simulink model "InverterComm2015"  (Simulink 8.1)
settings: Solver=ode45  StartTime=0.0  StopTime=10.0  RelTol=1e-3
libraries: simulink x24
settings Model: Creator=Brian  LastModifiedBy=Brian
settings DataIOCC: SignalLoggingSaveFormat=Dataset
settings OptimizationCC: ExpressionDepthLimit=128
settings DebuggingCC: FcnCallInpInsideContextMsg=EnableAllAsError
settings GRTTargetCC: CombineOutputUpdateFcns=on  GRTInterface=off

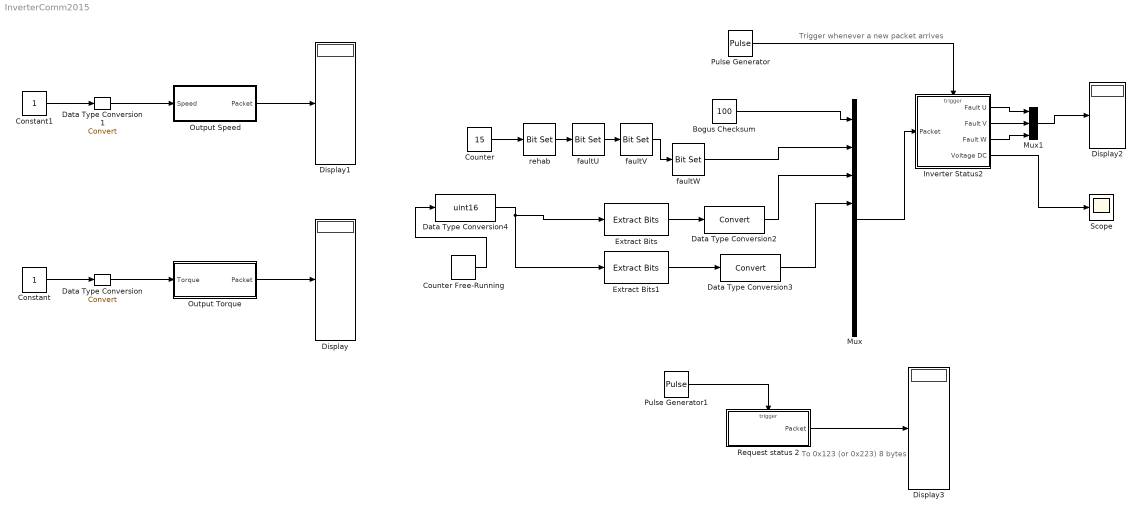
== system InverterComm2015 ==
  note: To 0x123 (or 0x223)
      | 8 bytes
  note: Trigger whenever a new packet arrives
  Bogus Checksum : Constant  Value=100  OutDataTypeStr=uint8
  Constant : Constant
  Constant1 : Constant
  Counter : Constant  Value=15  OutDataTypeStr=uint8
  Counter Free-Running : simulink/Sources/Counter Free-Running  NumBits=4  tsamp=-1
  Data Type Conversion : DataTypeConversion
  Data Type Conversion1 : DataTypeConversion
  Data Type Conversion2 : DataTypeConversion  ConvertRealWorld=Stored Integer (SI)
  Data Type Conversion3 : DataTypeConversion  ConvertRealWorld=Stored Integer (SI)
  Data Type Conversion4 : DataTypeConversion  OutDataTypeStr=uint16  ConvertRealWorld=Stored Integer (SI)
  Display{,1..3} (4 alike) : Display
      settings: Format=hex (Stored Integer)
  Extract Bits : simulink/Logic and Bit Operations/Extract Bits  bitsToExtract=Upper half  numBits=8  bitIdxRange=[0 7]  outScalingMode=Preserve fixed-point scaling
  Extract Bits1 : simulink/Logic and Bit Operations/Extract Bits  bitsToExtract=Lower half  numBits=8  bitIdxRange=[0 7]  outScalingMode=Preserve fixed-point scaling
  Inverter Status2 : Subsystem
  Mux : Mux  Inputs=8
  Mux1 : Mux  Inputs=3
  Output Speed : Subsystem
  Output Torque : Subsystem
  Pulse Generator : DiscretePulseGenerator  PulseType=Time based  Period=.1  PulseWidth=5
  Pulse Generator1 : DiscretePulseGenerator  PulseType=Time based  Period=.1  PulseWidth=5
  Request status 2 : Subsystem
  Scope : Scope
  faultU : simulink/Logic and Bit Operations/Bit Set  iBit=5
  faultV : simulink/Logic and Bit Operations/Bit Set  iBit=6
  faultW : simulink/Logic and Bit Operations/Bit Set  iBit=7
  rehab : simulink/Logic and Bit Operations/Bit Set  iBit=4
  wires:
  Output Torque/1(Packet) -> Display/1
  Constant/1 -> Data Type Conversion/1
  Data Type Conversion/1 -> Output Torque/1(Torque)
  Output Speed/1(Packet) -> Display1/1
  Constant1/1 -> Data Type Conversion1/1
  Data Type Conversion1/1 -> Output Speed/1(Speed)
  Pulse Generator/1 -> Inverter Status2/Trigger
  Mux/1 -> Inverter Status2/1(Packet)
  Bogus Checksum/1 -> Mux/1
  Counter/1 -> rehab/1
  rehab/1 -> faultU/1
  faultU/1 -> faultV/1
  faultV/1 -> faultW/1
  faultW/1 -> Mux/2
  Extract Bits/1 -> Data Type Conversion2/1
  Extract Bits1/1 -> Data Type Conversion3/1
  Counter Free-Running/1 -> Data Type Conversion4/1
  Data Type Conversion2/1 -> Mux/3
  Data Type Conversion3/1 -> Mux/4
  Inverter Status2/1(Fault U) -> Mux1/1
  Inverter Status2/2(Fault V) -> Mux1/2
  Inverter Status2/3(Fault W) -> Mux1/3
  Mux1/1 -> Display2/1
  Inverter Status2/4(Voltage DC) -> Scope/1
  Data Type Conversion4/1 -> Extract Bits1/1, Extract Bits/1
  Request status 2/1(Packet) -> Display3/1
  Pulse Generator1/1 -> Request status 2/Trigger

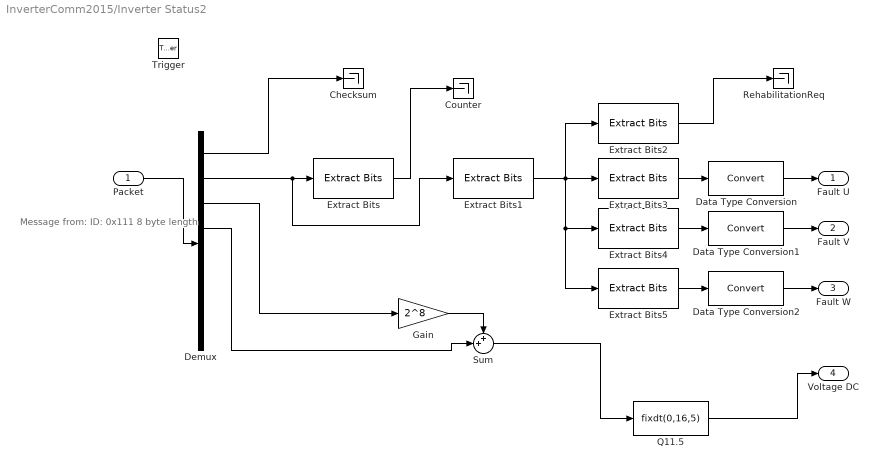
== system InverterComm2015/Inverter Status2 ==
  note: Message from:
      | ID: 0x111
      | 8 byte length
  Packet : Inport  OutDataTypeStr=uint8  PortDimensions=8
  Trigger : TriggerPort  PortDimensions=1
  Checksum : Terminator
  Counter : Terminator
  Data Type Conversion : DataTypeConversion
  Data Type Conversion1 : DataTypeConversion
  Data Type Conversion2 : DataTypeConversion
  Demux : Demux  Outputs=8
  Extract Bits : simulink/Logic and Bit Operations/Extract Bits  bitsToExtract=Lower half  numBits=8  bitIdxRange=[0 7]  outScalingMode=Treat bit field as an integer
  Extract Bits1 : simulink/Logic and Bit Operations/Extract Bits  bitsToExtract=Upper half  numBits=8  bitIdxRange=[0 7]  outScalingMode=Treat bit field as an integer
  Extract Bits2 : simulink/Logic and Bit Operations/Extract Bits  bitsToExtract=Range of bits  numBits=8  bitIdxRange=[0 0]  outScalingMode=Treat bit field as an integer
  Extract Bits3 : simulink/Logic and Bit Operations/Extract Bits  bitsToExtract=Range of bits  numBits=8  bitIdxRange=[1 1]  outScalingMode=Treat bit field as an integer
  Extract Bits4 : simulink/Logic and Bit Operations/Extract Bits  bitsToExtract=Range of bits  numBits=8  bitIdxRange=[2 2]  outScalingMode=Treat bit field as an integer
  Extract Bits5 : simulink/Logic and Bit Operations/Extract Bits  bitsToExtract=Range of bits  numBits=8  bitIdxRange=[3 3]  outScalingMode=Treat bit field as an integer
  Gain : Gain  Gain=2^8
  Q11.5 : DataTypeConversion  OutDataTypeStr=fixdt(0,16,5)
  RehabilitationReq : Terminator
  Sum : Sum  Inputs=++|
  Fault U : Outport  OutDataTypeStr=boolean
  Fault V : Outport  Port=2  OutDataTypeStr=boolean
  Fault W : Outport  Port=3  OutDataTypeStr=boolean
  Voltage DC : Outport  Port=4
  wires:
  Packet/1 -> Demux/1
  Demux/1 -> Checksum/1
  Demux/2 -> Extract Bits1/1, Extract Bits/1
  Extract Bits/1 -> Counter/1
  Extract Bits1/1 -> Extract Bits2/1, Extract Bits5/1, Extract Bits4/1, Extract Bits3/1
  Extract Bits2/1 -> RehabilitationReq/1
  Extract Bits3/1 -> Data Type Conversion/1
  Extract Bits4/1 -> Data Type Conversion1/1
  Extract Bits5/1 -> Data Type Conversion2/1
  Data Type Conversion/1 -> Fault U/1
  Data Type Conversion1/1 -> Fault V/1
  Data Type Conversion2/1 -> Fault W/1
  Demux/3 -> Gain/1
  Gain/1 -> Sum/1
  Sum/1 -> Q11.5/1
  Demux/4 -> Sum/2
  Q11.5/1 -> Voltage DC/1

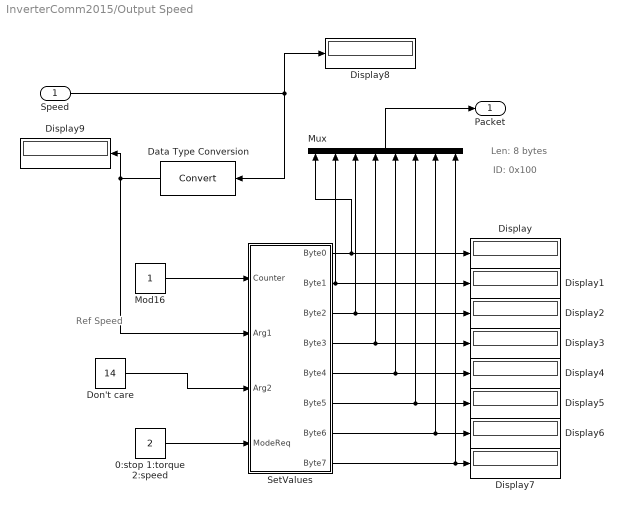
== system InverterComm2015/Output Speed ==
  note: ID: 0x100
  note: Len: 8 bytes
  note: Ref
      | Speed
  Speed : Inport  OutDataTypeStr=single
  0:stop 1:torque 2:speed : Constant  Value=2  OutDataTypeStr=uint8
  Data Type Conversion : DataTypeConversion
  Display{,1..9} (10 alike) : Display
  Don't care : Constant  Value=14  OutDataTypeStr=fixdt(1,16,5)
  Mod16 : Constant  OutDataTypeStr=uint8
  Mux : Mux  Inputs=8
  SetValues : Subsystem
  Packet : Outport
  wires:
  Data Type Conversion/1 -> Display9/1, SetValues/2(Arg1)
  Mux/1 -> Packet/1
  SetValues/8(Byte7) -> Display7/1, Mux/8
  SetValues/7(Byte6) -> Display6/1, Mux/7
  SetValues/6(Byte5) -> Mux/6, Display5/1
  SetValues/5(Byte4) -> Mux/5, Display4/1
  SetValues/4(Byte3) -> Mux/4, Display3/1
  SetValues/3(Byte2) -> Mux/3, Display2/1
  SetValues/2(Byte1) -> Mux/2, Display1/1
  SetValues/1(Byte0) -> Display/1, Mux/1
  Don't care/1 -> SetValues/3(Arg2)
  Speed/1 -> Display8/1, Data Type Conversion/1
  Mod16/1 -> SetValues/1(Counter)
  0:stop 1:torque 2:speed/1 -> SetValues/4(ModeReq)

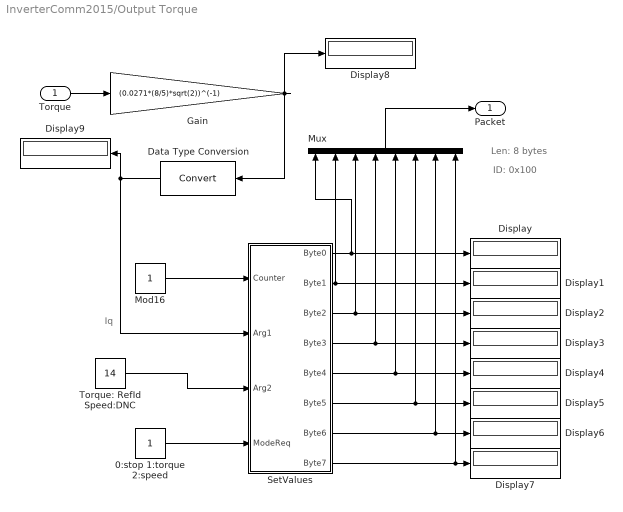
== system InverterComm2015/Output Torque ==
  note: Iq
  note: Len: 8 bytes
  note: ID: 0x100
  Torque : Inport  OutDataTypeStr=single
  0:stop 1:torque 2:speed : Constant  OutDataTypeStr=uint8
  Data Type Conversion : DataTypeConversion
  Display{,1..9} (10 alike) : Display
  Gain : Gain  Gain=(0.0271*(8/5)*sqrt(2))^(-1)
  Mod16 : Constant  OutDataTypeStr=uint8
  Mux : Mux  Inputs=8
  SetValues : Subsystem
  Torque: RefId Speed:DNC : Constant  Value=14  OutDataTypeStr=fixdt(1,16,5)
  Packet : Outport
  wires:
  0:stop 1:torque 2:speed/1 -> SetValues/4(ModeReq)
  Mod16/1 -> SetValues/1(Counter)
  Gain/1 -> Data Type Conversion/1, Display8/1
  Torque: RefId Speed:DNC/1 -> SetValues/3(Arg2)
  SetValues/1(Byte0) -> Mux/1, Display/1
  SetValues/2(Byte1) -> Display1/1, Mux/2
  SetValues/3(Byte2) -> Display2/1, Mux/3
  SetValues/4(Byte3) -> Display3/1, Mux/4
  SetValues/5(Byte4) -> Display4/1, Mux/5
  SetValues/6(Byte5) -> Display5/1, Mux/6
  SetValues/7(Byte6) -> Mux/7, Display6/1
  SetValues/8(Byte7) -> Mux/8, Display7/1
  Mux/1 -> Packet/1
  Torque/1 -> Gain/1
  Data Type Conversion/1 -> SetValues/2(Arg1), Display9/1

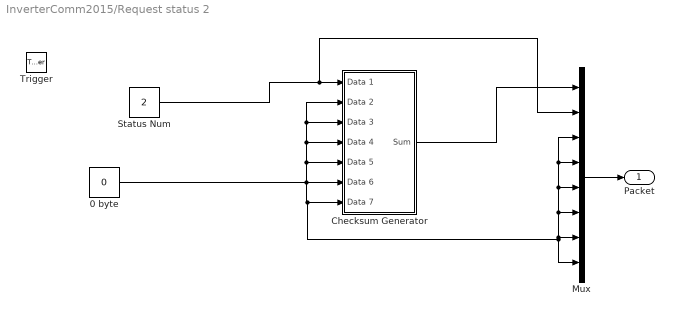
== system InverterComm2015/Request status 2 ==
  Trigger : TriggerPort  PortDimensions=1
  0 byte : Constant  Value=0  OutDataTypeStr=uint8
  Checksum Generator : Subsystem
  Mux : Mux  Inputs=8
  Status Num : Constant  Value=2  OutDataTypeStr=uint8
  Packet : Outport
  wires:
  Status Num/1 -> Mux/2, Checksum Generator/1(Data 1)
  Mux/1 -> Packet/1
  Checksum Generator/1(Sum) -> Mux/1
  0 byte/1 -> Mux/7, Mux/6, Mux/5, Mux/4, Mux/3, Mux/8, Checksum Generator/7(Data 7), Checksum Generator/6(Data 6), Checksum Generator/5(Data 5), Checksum Generator/4(Data 4), Checksum Generator/3(Data 3), Checksum Generator/2(Data 2)

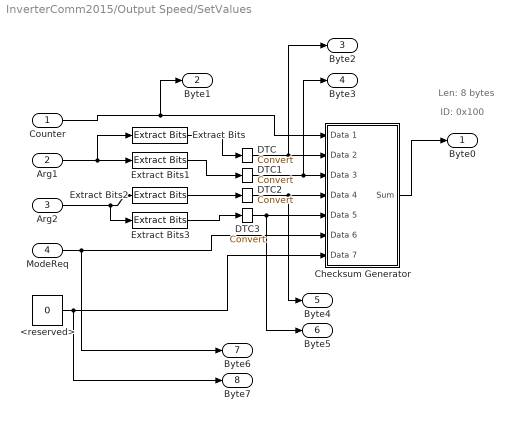
== system InverterComm2015/Output Speed/SetValues ==
  note: ID: 0x100
  note: Len: 8 bytes
  Counter : Inport  OutDataTypeStr=uint8
  Arg1 : Inport  Port=2  OutDataTypeStr=fixdt(1,16,1)
  Arg2 : Inport  Port=3  OutDataTypeStr=fixdt(1,16,5)  LockScale=on
  ModeReq : Inport  Port=4  OutDataTypeStr=uint8
  <reserved> : Constant  Value=0  OutDataTypeStr=uint8
  Checksum Generator : Subsystem
  DTC{,1..3} (4 alike) : DataTypeConversion  ConvertRealWorld=Stored Integer (SI)
  Extract Bits : simulink/Logic and Bit Operations/Extract Bits  bitsToExtract=Upper half  numBits=8  bitIdxRange=[0 7]  outScalingMode=Treat bit field as an integer
  Extract Bits1 : simulink/Logic and Bit Operations/Extract Bits  bitsToExtract=Lower half  numBits=8  bitIdxRange=[0 7]  outScalingMode=Treat bit field as an integer
  Extract Bits2 : simulink/Logic and Bit Operations/Extract Bits  bitsToExtract=Upper half  numBits=8  bitIdxRange=[0 7]  outScalingMode=Treat bit field as an integer
  Extract Bits3 : simulink/Logic and Bit Operations/Extract Bits  bitsToExtract=Lower half  numBits=8  bitIdxRange=[0 7]  outScalingMode=Treat bit field as an integer
  Byte0 : Outport
  Byte1 : Outport  Port=2
  Byte2 : Outport  Port=3
  Byte3 : Outport  Port=4
  Byte4 : Outport  Port=5
  Byte5 : Outport  Port=6
  Byte6 : Outport  Port=7
  Byte7 : Outport  Port=8
  wires:
  DTC3/1 -> Checksum Generator/5(Data 5), Byte5/1
  DTC2/1 -> Checksum Generator/4(Data 4), Byte4/1
  DTC1/1 -> Checksum Generator/3(Data 3), Byte3/1
  DTC/1 -> Checksum Generator/2(Data 2), Byte2/1
  Checksum Generator/1(Sum) -> Byte0/1
  <reserved>/1 -> Byte7/1, Checksum Generator/7(Data 7)
  ModeReq/1 -> Checksum Generator/6(Data 6), Byte6/1
  Extract Bits3/1 -> DTC3/1
  Extract Bits2/1 -> DTC2/1
  Extract Bits1/1 -> DTC1/1
  Extract Bits/1 -> DTC/1
  Counter/1 -> Checksum Generator/1(Data 1), Byte1/1
  Arg2/1 -> Extract Bits2/1, Extract Bits3/1
  Arg1/1 -> Extract Bits/1, Extract Bits1/1

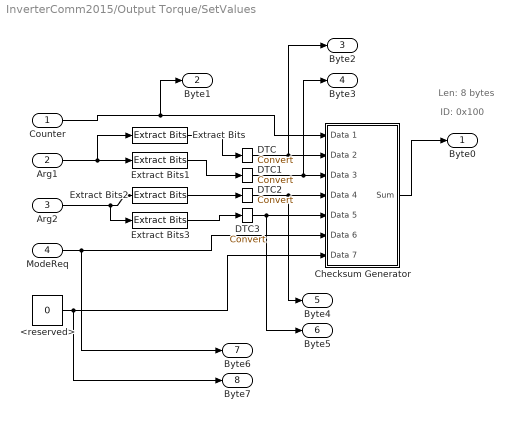
== system InverterComm2015/Output Torque/SetValues ==
  note: Len: 8 bytes
  note: ID: 0x100
  Counter : Inport  OutDataTypeStr=uint8
  Arg1 : Inport  Port=2  OutDataTypeStr=fixdt(1,16,5)
  Arg2 : Inport  Port=3  OutDataTypeStr=fixdt(1,16,5)  LockScale=on
  ModeReq : Inport  Port=4  OutDataTypeStr=uint8
  <reserved> : Constant  Value=0  OutDataTypeStr=uint8
  Checksum Generator : Subsystem
  DTC{,1..3} (4 alike) : DataTypeConversion  ConvertRealWorld=Stored Integer (SI)
  Extract Bits : simulink/Logic and Bit Operations/Extract Bits  bitsToExtract=Upper half  numBits=8  bitIdxRange=[0 7]  outScalingMode=Treat bit field as an integer
  Extract Bits1 : simulink/Logic and Bit Operations/Extract Bits  bitsToExtract=Lower half  numBits=8  bitIdxRange=[0 7]  outScalingMode=Treat bit field as an integer
  Extract Bits2 : simulink/Logic and Bit Operations/Extract Bits  bitsToExtract=Upper half  numBits=8  bitIdxRange=[0 7]  outScalingMode=Treat bit field as an integer
  Extract Bits3 : simulink/Logic and Bit Operations/Extract Bits  bitsToExtract=Lower half  numBits=8  bitIdxRange=[0 7]  outScalingMode=Treat bit field as an integer
  Byte0 : Outport
  Byte1 : Outport  Port=2
  Byte2 : Outport  Port=3
  Byte3 : Outport  Port=4
  Byte4 : Outport  Port=5
  Byte5 : Outport  Port=6
  Byte6 : Outport  Port=7
  Byte7 : Outport  Port=8
  wires:
  Arg1/1 -> Extract Bits1/1, Extract Bits/1
  Arg2/1 -> Extract Bits3/1, Extract Bits2/1
  Counter/1 -> Byte1/1, Checksum Generator/1(Data 1)
  Extract Bits/1 -> DTC/1
  Extract Bits1/1 -> DTC1/1
  Extract Bits2/1 -> DTC2/1
  Extract Bits3/1 -> DTC3/1
  ModeReq/1 -> Byte6/1, Checksum Generator/6(Data 6)
  <reserved>/1 -> Checksum Generator/7(Data 7), Byte7/1
  Checksum Generator/1(Sum) -> Byte0/1
  DTC/1 -> Byte2/1, Checksum Generator/2(Data 2)
  DTC1/1 -> Byte3/1, Checksum Generator/3(Data 3)
  DTC2/1 -> Byte4/1, Checksum Generator/4(Data 4)
  DTC3/1 -> Byte5/1, Checksum Generator/5(Data 5)

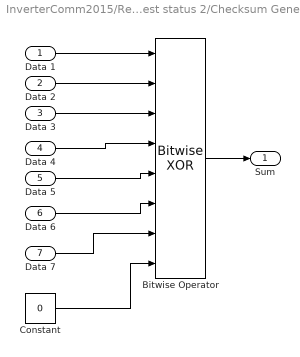
== system InverterComm2015/Request status 2/Checksum Generator ==
  Data 1 : Inport
  Data 2 : Inport  Port=2
  Data 3 : Inport  Port=3
  Data 4 : Inport  Port=4
  Data 5 : Inport  Port=5
  Data 6 : Inport  Port=6
  Data 7 : Inport  Port=7
  Bitwise Operator : simulink/Logic and Bit Operations/Bitwise Operator  logicop=XOR  UseBitMask=off  NumInputPorts=8  BitMask=bin2dec('11011001')  BitMaskRealWorld=Stored Integer
  Constant : Constant  Value=0  OutDataTypeStr=uint8
  Sum : Outport  OutDataTypeStr=uint8
  wires:
  Data 1/1 -> Bitwise Operator/1
  Data 2/1 -> Bitwise Operator/2
  Data 3/1 -> Bitwise Operator/3
  Data 4/1 -> Bitwise Operator/4
  Data 5/1 -> Bitwise Operator/5
  Data 6/1 -> Bitwise Operator/6
  Data 7/1 -> Bitwise Operator/7
  Constant/1 -> Bitwise Operator/8
  Bitwise Operator/1 -> Sum/1

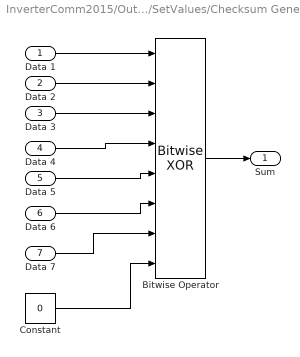
== system InverterComm2015/Output Speed/SetValues/Checksum Generator ==
  Data 1 : Inport
  Data 2 : Inport  Port=2
  Data 3 : Inport  Port=3
  Data 4 : Inport  Port=4
  Data 5 : Inport  Port=5
  Data 6 : Inport  Port=6
  Data 7 : Inport  Port=7
  Bitwise Operator : simulink/Logic and Bit Operations/Bitwise Operator  logicop=XOR  UseBitMask=off  NumInputPorts=8  BitMask=bin2dec('11011001')  BitMaskRealWorld=Stored Integer
  Constant : Constant  Value=0  OutDataTypeStr=uint8
  Sum : Outport  OutDataTypeStr=uint8
  wires:
  Bitwise Operator/1 -> Sum/1
  Constant/1 -> Bitwise Operator/8
  Data 7/1 -> Bitwise Operator/7
  Data 6/1 -> Bitwise Operator/6
  Data 5/1 -> Bitwise Operator/5
  Data 4/1 -> Bitwise Operator/4
  Data 3/1 -> Bitwise Operator/3
  Data 2/1 -> Bitwise Operator/2
  Data 1/1 -> Bitwise Operator/1

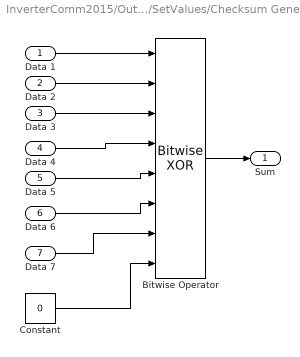
== system InverterComm2015/Output Torque/SetValues/Checksum Generator ==
  Data 1 : Inport
  Data 2 : Inport  Port=2
  Data 3 : Inport  Port=3
  Data 4 : Inport  Port=4
  Data 5 : Inport  Port=5
  Data 6 : Inport  Port=6
  Data 7 : Inport  Port=7
  Bitwise Operator : simulink/Logic and Bit Operations/Bitwise Operator  logicop=XOR  UseBitMask=off  NumInputPorts=8  BitMask=bin2dec('11011001')  BitMaskRealWorld=Stored Integer
  Constant : Constant  Value=0  OutDataTypeStr=uint8
  Sum : Outport  OutDataTypeStr=uint8
  wires:
  Data 1/1 -> Bitwise Operator/1
  Data 2/1 -> Bitwise Operator/2
  Data 3/1 -> Bitwise Operator/3
  Data 4/1 -> Bitwise Operator/4
  Data 5/1 -> Bitwise Operator/5
  Data 6/1 -> Bitwise Operator/6
  Data 7/1 -> Bitwise Operator/7
  Constant/1 -> Bitwise Operator/8
  Bitwise Operator/1 -> Sum/1
